simulink model "DYN_6DOF"  (R2018b)
(part 17 of 18)

(m6*the5_dot*x6*z6*cos(the6))/2 + (m6*the5_dot*y6*z6*sin(the6))/2 + (IPy6*the2_dot*cos(the5)*cos(the6)*sin(the4))/2 + (IPy6*the3_dot*cos(the5)*cos(the6)*sin(the4))/2 + (IPz6*the2_dot*cos(the5)*sin(the4)*sin(the6))/2 + (IPz6*the3_dot*cos(the5)*sin(the4)*sin(the6))/2 - (m6*the4_dot*x6*z6*sin(the5)*sin(the6))/2 + (IPy6*the1_dot*cos(the2)*cos(the3)*cos(the6)*sin(the5))/2 + (IPz6*the1_dot*cos(the2)*cos(the6)*sin(the3)*sin(the4))/2 + (IPz6*the1_dot*cos(the3)*cos(the6)*sin(the2)*sin(the4))/2 + (IPz6*the1_dot*cos(the2)*cos(the3)*sin(the5)*sin(the6))/2 - (IPy6*the1_dot*cos(the2)*sin(the3)*sin(the4)*sin(the6))/2 - (IPy6*the1_dot*cos(the3)*sin(the2)*sin(the4)*sin(the6))/2 - (IPy6*the1_dot*cos(the6)*sin(the2)*sin(the3)*sin(the5))/2 - (IPz6*the1_dot*sin(the2)*sin(the3)*sin(the5)*sin(the6))/2 - (a1*m6*the1_dot*y6*cos(the4)*cos(the6))/2 - (a1*m6*the1_dot*x6*cos(the4)*sin(the6))/2 + (a3*m6*the2_dot*x6*cos(the6)*sin(the5))/2 + (a3*m6*the3_dot*x6*cos(the6)*sin(the5))/2 + (d4*m6*the2_dot*y6*cos(the6)*sin(the4))/2 + (d4*m6*the3_dot*y6*cos(the6)*sin(the4))/2 - (m6*the2_dot*x6*z6*cos(the4)*cos(the6))/2 - (m6*the3_dot*x6*z6*cos(the4)*cos(the6))/2 - (a3*m6*the2_dot*y6*sin(the5)*sin(the6))/2 - (a3*m6*the3_dot*y6*sin(the5)*sin(the6))/2 + (d4*m6*the2_dot*x6*sin(the4)*sin(the6))/2 + (d4*m6*the3_dot*x6*sin(the4)*sin(the6))/2 + (m6*the2_dot*y6*z6*cos(the4)*sin(the6))/2 + (m6*the3_dot*y6*z6*cos(the4)*sin(the6))/2 - (m6*the4_dot*y6*z6*cos(the6)*sin(the5))/2 + (IPy6*the1_dot*cos(the2)*cos(the4)*cos(the5)*cos(the6)*sin(the3))/2 + (IPy6*the1_dot*cos(the3)*cos(the4)*cos(the5)*cos(the6)*sin(the2))/2 + (IPz6*the1_dot*cos(the2)*cos(the4)*cos(the5)*sin(the3)*sin(the6))/2 + (IPz6*the1_dot*cos(the3)*cos(the4)*cos(the5)*sin(the2)*sin(the6))/2 - (a2*m6*the1_dot*y6*cos(the2)*cos(the4)*cos(the6))/2 - (d4*m6*the2_dot*x6*cos(the4)*cos(the5)*cos(the6))/2 - (d4*m6*the3_dot*x6*cos(the4)*cos(the5)*cos(the6))/2 - (a2*m6*the1_dot*x6*cos(the2)*cos(the4)*sin(the6))/2 - (a1*m6*the1_dot*x6*cos(the5)*cos(the6)*sin(the4))/2 + (a2*m6*the2_dot*x6*cos(the3)*cos(the6)*sin(the5))/2 + (d4*m6*the2_dot*y6*cos(the4)*cos(the5)*sin(the6))/2 + (d4*m6*the3_dot*y6*cos(the4)*cos(the5)*sin(the6))/2 + (a1*m6*the1_dot*y6*cos(the5)*sin(the4)*sin(the6))/2 - (a2*m6*the2_dot*y6*cos(the6)*sin(the3)*sin(the4))/2 - (a2*m6*the2_dot*y6*cos(the3)*sin(the5)*sin(the6))/2 + (m6*the2_dot*y6*z6*cos(the5)*cos(the6)*sin(the4))/2 + (m6*the3_dot*y6*z6*cos(the5)*cos(the6)*sin(the4))/2 - (a2*m6*the2_dot*x6*sin(the3)*sin(the4)*sin(the6))/2 + (m6*the2_dot*x6*z6*cos(the5)*sin(the4)*sin(the6))/2 + (m6*the3_dot*x6*z6*cos(the5)*sin(the4)*sin(the6))/2 - (a3*m6*the1_dot*y6*cos(the2)*cos(the3)*cos(the4)*cos(the6))/2 - (a3*m6*the1_dot*x6*cos(the2)*cos(the3)*cos(the4)*sin(the6))/2 - (a2*m6*the1_dot*x6*cos(the2)*cos(the5)*cos(the6)*sin(the4))/2 + (a2*m6*the2_dot*x6*cos(the4)*cos(the5)*cos(the6)*sin(the3))/2 + (d4*m6*the1_dot*y6*cos(the2)*cos(the4)*cos(the6)*sin(the3))/2 + (d4*m6*the1_dot*y6*cos(the3)*cos(the4)*cos(the6)*sin(the2))/2 + (a3*m6*the1_dot*y6*cos(the4)*cos(the6)*sin(the2)*sin(the3))/2 + (a2*m6*the1_dot*y6*cos(the2)*cos(the5)*sin(the4)*sin(the6))/2 - (a2*m6*the2_dot*y6*cos(the4)*cos(the5)*sin(the3)*sin(the6))/2 + (d4*m6*the1_dot*x6*cos(the2)*cos(the4)*sin(the3)*sin(the6))/2 + (d4*m6*the1_dot*x6*cos(the3)*cos(the4)*sin(the2)*sin(the6))/2 + (m6*the1_dot*y6*z6*cos(the2)*cos(the3)*cos(the6)*sin(the5))/2 + (a3*m6*the1_dot*x6*cos(the4)*sin(the2)*sin(the3)*sin(the6))/2 + (m6*the1_dot*x6*z6*cos(the2)*cos(the6)*sin(the3)*sin(the4))/2 + (m6*the1_dot*x6*z6*cos(the3)*cos(the6)*sin(the2)*sin(the4))/2 + (m6*the1_dot*x6*z6*cos(the2)*cos(the3)*sin(the5)*sin(the6))/2 - (m6*the1_dot*y6*z6*cos(the2)*sin(the3)*sin(the4)*sin(the6))/2 - (m6*the1_dot*y6*z6*cos(the3)*sin(the2)*sin(the4)*sin(the6))/2 - (m6*the1_dot*y6*z6*cos(the6)*sin(the2)*sin(the3)*sin(the5))/2 - (m6*the1_dot*x6*z6*sin(the2)*sin(the3)*sin(the5)*sin(the6))/2 - (a3*m6*the1_dot*x6*cos(the2)*cos(the3)*cos(the5)*cos(the6)*sin(the4))/2 + (a3*m6*the1_dot*y6*cos(the2)*cos(the3)*cos(the5)*sin(the4)*sin(the6))/2 + (d4*m6*the1_dot*x6*cos(the2)*cos(the5)*cos(the6)*sin(the3)*sin(the4))/2 + (d4*m6*the1_dot*x6*cos(the3)*cos(the5)*cos(the6)*sin(the2)*sin(the4))/2 + (m6*the1_dot*y6*z6*cos(the2)*cos(the4)*cos(the5)*cos(the6)*sin(the3))/2 + (m6*the1_dot*y6*z6*cos(the3)*cos(the4)*cos(the5)*cos(the6)*sin(the2))/2 + (a3*m6*the1_dot*x6*cos(the5)*cos(the6)*sin(the2)*sin(the3)*sin(the4))/2 - (d4*m6*the1_dot*y6*cos(the2)*cos(the5)*sin(the3)*sin(the4)*sin(the6))/2 - (d4*m6*the1_dot*y6*cos(the3)*cos(the5)*sin(the2)*sin(the4)*sin(the6))/2 + (m6*the1_dot*x6*z6*cos(the2)*cos(the4)*cos(the5)*sin(the3)*sin(the6))/2 + (m6*the1_dot*x6*z6*cos(the3)*cos(the4)*cos(the5)*sin(the2)*sin(the6))/2 - (a3*m6*the1_dot*y6*cos(the5)*sin(the2)*sin(the3)*sin(the4)*sin(the6))/2];

G=...
[0;
-g*(m3*y3*sin(the2 + the3) + m4*z4*sin(the2 + the3) - a2*m3*cos(the2) - a2*m4*cos(the2) - a2*m5*cos(the2) - a2*m6*cos(the2) - m2*x2*cos(the2) + m2*y2*sin(the2) - a3*m4*cos(the2 + the3) - a3*m5*cos(the2 + the3) - a3*m6*cos(the2 + the3) + d4*m4*sin(the2 + the3) + d4*m5*sin(the2 + the3) + d4*m6*sin(the2 + the3) - m3*x3*cos(the2 + the3) - m4*x4*cos(the2 + the3)*cos(the4) + m4*y4*cos(the2 + the3)*sin(the4) + m5*y5*sin(the2 + the3)*cos(the5) - m5*z5*cos(the2 + the3)*sin(the4) + m6*z6*sin(the2 + the3)*cos(the5) + m5*x5*sin(the2 + the3)*sin(the5) - m5*x5*cos(the2 + the3)*cos(the4)*cos(the5) + m5*y5*cos(the2 + the3)*cos(the4)*sin(the5) + m6*y6*cos(the2 + the3)*cos(the6)*sin(the4) + m6*z6*cos(the2 + the3)*cos(the4)*sin(the5) + m6*x6*cos(the2 + the3)*sin(the4)*sin(the6) + m6*x6*sin(the2 + the3)*cos(the6)*sin(the5) - m6*y6*sin(the2 + the3)*sin(the5)*sin(the6) - m6*x6*cos(the2 + the3)*cos(the4)*cos(the5)*cos(the6) + m6*y6*cos(the2 + the3)*cos(the4)*cos(the5)*sin(the6));
-g*(m3*y3*sin(the2 + the3) + m4*z4*sin(the2 + the3) - a3*m4*cos(the2 + the3) - a3*m5*cos(the2 + the3) - a3*m6*cos(the2 + the3) + d4*m4*sin(the2 + the3) + d4*m5*sin(the2 + the3) + d4*m6*sin(the2 + the3) - m3*x3*cos(the2 + the3) - m4*x4*cos(the2 + the3)*cos(the4) + m4*y4*cos(the2 + the3)*sin(the4) + m5*y5*sin(the2 + the3)*cos(the5) - m5*z5*cos(the2 + the3)*sin(the4) + m6*z6*sin(the2 + the3)*cos(the5) + m5*x5*sin(the2 + the3)*sin(the5) - m5*x5*cos(the2 + the3)*cos(the4)*cos(the5) + m5*y5*cos(the2 + the3)*cos(the4)*sin(the5) + m6*y6*cos(the2 + the3)*cos(the6)*sin(the4) + m6*z6*cos(the2 + the3)*cos(the4)*sin(the5) + m6*x6*cos(the2 + the3)*sin(the4)*sin(the6) + m6*x6*sin(the2 + the3)*cos(the6)*sin(the5) - m6*y6*sin(the2 + the3)*sin(the5)*sin(the6) - m6*x6*cos(the2 + the3)*cos(the4)*cos(the5)*cos(the6) + m6*y6*cos(the2 + the3)*cos(the4)*cos(the5)*sin(the6));
-g*(m4*y4*sin(the2 + the3)*cos(the4) - m5*z5*sin(the2 + the3)*cos(the4) + m4*x4*sin(the2 + the3)*sin(the4) + m6*y6*sin(the2 + the3)*cos(the4)*cos(the6) + m5*x5*sin(the2 + the3)*cos(the5)*sin(the4) + m6*x6*sin(the2 + the3)*cos(the4)*sin(the6) - m5*y5*sin(the2 + the3)*sin(the4)*sin(the5) - m6*z6*sin(the2 + the3)*sin(the4)*sin(the5) + m6*x6*sin(the2 + the3)*cos(the5)*cos(the6)*sin(the4) - m6*y6*sin(the2 + the3)*cos(the5)*sin(the4)*sin(the6));
-g*(m5*y5*cos(the2 + the3)*sin(the5) - m5*x5*cos(the2 + the3)*cos(the5) + m6*z6*cos(the2 + the3)*sin(the5) - m6*x6*cos(the2 + the3)*cos(the5)*cos(the6) + m5*y5*sin(the2 + the3)*cos(the4)*cos(the5) + m6*y6*cos(the2 + the3)*cos(the5)*sin(the6) + m6*z6*sin(the2 + the3)*cos(the4)*cos(the5) + m5*x5*sin(the2 + the3)*cos(the4)*sin(the5) + m6*x6*sin(the2 + the3)*cos(the4)*cos(the6)*sin(the5) - m6*y6*sin(the2 + the3)*cos(the4)*sin(the5)*sin(the6));
-g*(m6*y6*cos(the2 + the3)*cos(the6)*sin(the5) + m6*x6*sin(the2 + the3)*cos(the6)*sin(the4) + m6*x6*cos(the2 + the3)*sin(the5)*sin(the6) - m6*y6*sin(the2 + the3)*sin(the4)*sin(the6) + m6*y6*sin(the2 + the3)*cos(the4)*cos(the5)*cos(the6) + m6*x6*sin(the2 + the3)*cos(the4)*cos(the5)*sin(the6))];
